simulink model "Controllo_assey_4gdl"  (R2020b)
settings: Solver=VariableStepAuto  StartTime=0.0  StopTime=3  RelTol=1e-3
values from neighbouring files (symbols this model uses):
  my = config_dc(pary)    [mainy.m]
  pary = parametriy ()    [mainy.m]
undefined symbols (not defined in the file or in its folder): accelerazioniy, Evaluate_Trajectory
libraries: cstblocks x4
settings Model: Creator=stefa  LastModifiedBy=user
settings DebuggingCC: SFMachineParentedDataDiag=error

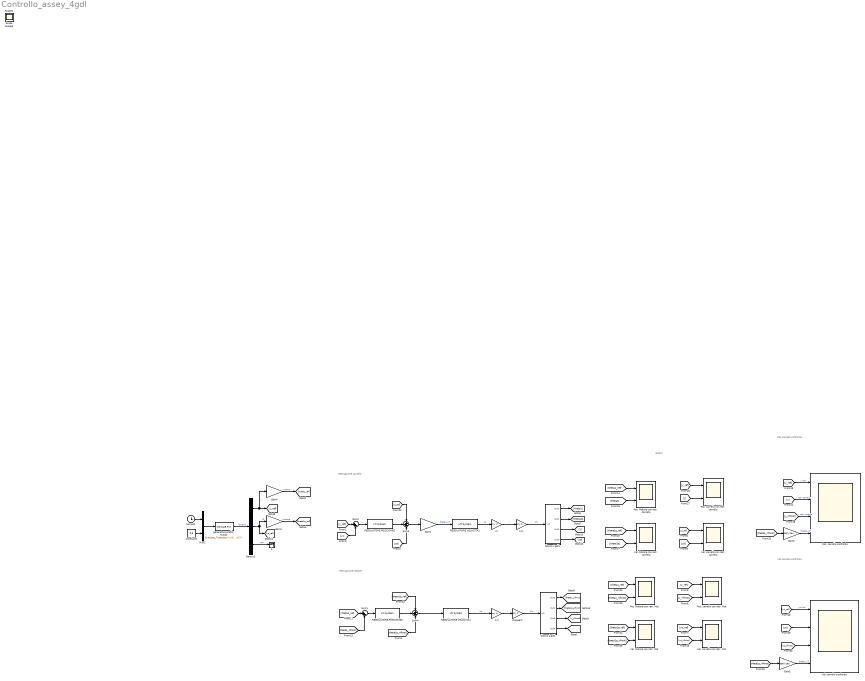
== system Controllo_assey_4gdl ==
  note: Retroazione carrello
  note: Retroazione Motore
  note: Grafici
  note: Pos carrello confronto
  note: Vel carrello confronto
  " 1" : Terminator
  Constant1 : Constant  Value=0.6
  Demux2 : Demux  Outputs=3
  Gain1 : Gain  Gain=1/pary.tau
  Gain2 : Gain  Gain=1/pary.tau
  Gain3 : Gain  Gain=pary.tau
  Gain4 : Gain  Gain=1/pary.tau
  Gain5 : Gain  Gain=pary.tau
  Km : Gain  Gain=my.K
  Kr : Gain  Gain=my.Kr
  Kr1 : Gain  Gain=my.Kr
  Mux1 : Mux  Inputs=2
  Pos. Motore con retr. Mot : Scope  NumInputPorts=2
  Pos. Motore con retr. carrello : Scope  NumInputPorts=2
  Pos. carrello con retr. Mot : Scope  NumInputPorts=2
  Pos. carrello con retr. carrello : Scope  NumInputPorts=2
  Pos. carrello confronto : Scope  NumInputPorts=4
  REGOLATORE POSIZIONE1 : cstblocks/LTI System  sys=ap.H_P  IC=[]
  REGOLATORE POSIZIONE2 : cstblocks/LTI System  sys=ap.H_P  IC=[]
  REGOLATORE VELOCITA1 : cstblocks/LTI System  sys=av.PI_V  IC=[]
  REGOLATORE VELOCITA2 : cstblocks/LTI System  sys=av.PI_V  IC=[]
  Sum1 : Sum  Inputs=|+-
  Sum2 : Sum  Inputs=|+-
  Sum3 : Sum  Inputs=++-
  Sum4 : Sum  Inputs=++-
  Vel. Motore con retr. Mot : Scope  NumInputPorts=2
  Vel. Motore con retr. carrello : Scope  NumInputPorts=2
  Vel. carrello con retr. Mot : Scope  NumInputPorts=2
  Vel. carrello con retr. carrello : Scope  NumInputPorts=2
  Vel. carrello confronto : Scope  NumInputPorts=4
  blocco 4 gdl1 : Subsystem
  blocco 4 gdl2 : Subsystem
  chopper2 : Gain  Gain=my.K
  generatore profilo moto2 : MATLABFcn  MATLABFcn=Evaluate_Trajectory( u(1) , u(2))  OutputDimensions=3
  tempo2 : Clock
  Scope : Scope
  Scope1 : Scope
  Scope3 : Scope
  wires:
  Kr/1 -> Km/1  "I"
  REGOLATORE VELOCITA2/1 -> Kr/1  "Va"
  REGOLATORE POSIZIONE1/1 -> Sum3/2
  Demux2/3 -> " 1"/1  "YPP"
  Mux1/1 -> generatore profilo moto2/1
  generatore profilo moto2/1 -> Demux2/1  "carrello"
  Constant1/1 -> Mux1/2
  [yp_ref] -> Vel. carrello con retr. carrello/1
  [yp] -> Vel. carrello con retr. carrello/2
  [y_ref] -> Pos. carrello con retr. carrello/1
  [y] -> Pos. carrello con retr. carrello/2
  Sum2/1 -> REGOLATORE POSIZIONE1/1
  tempo2/1 -> Mux1/1
  blocco 4 gdl1/3(Out3) -> [y]
  blocco 4 gdl1/4(Out4) -> [yp]
  Km/1 -> blocco 4 gdl1/1(In1)  "Cm"
  Demux2/1 -> [y_ref], Gain4/1  "Y"
  Demux2/2 -> Gain1/1, [yp_ref]  "YP"
  [yp_ref] -> Sum3/1
  Sum3/1 -> Gain2/1
  Gain2/1 -> REGOLATORE VELOCITA2/1  "theta1_rif"
  blocco 4 gdl1/1(Out2) -> [theta1]
  blocco 4 gdl1/2(Out1) -> [theta1p]
  [y_ref] -> Sum2/1
  [y] -> Sum2/2
  [yp] -> Sum3/3
  blocco 4 gdl2/4(Out4) -> [yp_rifmot]
  [y_rifmot] -> Pos. carrello con retr. Mot/2
  chopper2/1 -> blocco 4 gdl2/1(In1)  "Cm"
  blocco 4 gdl2/3(Out3) -> [y_rifmot]
  [theta1_ref] -> Pos. Motore con retr. Mot/1
  Kr1/1 -> chopper2/1  "I"
  Sum1/1 -> REGOLATORE POSIZIONE2/1
  [theta1p_ref] -> Vel. Motore con retr. Mot/1
  REGOLATORE POSIZIONE2/1 -> Sum4/2
  REGOLATORE VELOCITA1/1 -> Kr1/1  "Va"
  blocco 4 gdl2/2(Out1) -> [theta1p_rifmot]
  blocco 4 gdl2/1(Out2) -> [theta1_rifmot]
  [yp_rifmot] -> Vel. carrello con retr. Mot/2
  [yp_ref] -> Vel. carrello con retr. Mot/1
  Sum4/1 -> REGOLATORE VELOCITA1/1
  [y_ref] -> Pos. carrello con retr. Mot/1
  [theta1p_rifmot] -> Vel. Motore con retr. Mot/2
  [theta1_rifmot] -> Pos. Motore con retr. Mot/2
  [theta1p_ref] -> Sum4/1
  Gain4/1 -> [theta1_ref]  "motore"
  [theta1_ref] -> Sum1/1
  Gain1/1 -> [theta1p_ref]  "motore"
  [theta1p_rifmot] -> Sum4/3
  [theta1_rifmot] -> Sum1/2
  [theta1p] -> Vel. Motore con retr. carrello/2
  [theta1] -> Pos. Motore con retr. carrello/2
  [theta1p_ref] -> Vel. Motore con retr. carrello/1
  [theta1_ref] -> Pos. Motore con retr. carrello/1
  [y] -> Pos. carrello confronto/2  "y retr. carrello"
  [y_ref] -> Pos. carrello confronto/1  "y ldm"
  [y_rifmot] -> Pos. carrello confronto/3  "y retr. motore"
  [yp] -> Vel. carrello confronto/2
  [yp_ref] -> Vel. carrello confronto/1  "yp ldm"
  [yp_rifmot] -> Vel. carrello confronto/3
  [theta1_rifmot] -> Gain3/1
  Gain3/1 -> Pos. carrello confronto/4  "theta1_rif"
  [theta1p_rifmot] -> Gain5/1
  Gain5/1 -> Vel. carrello confronto/4  "theta1_rif"

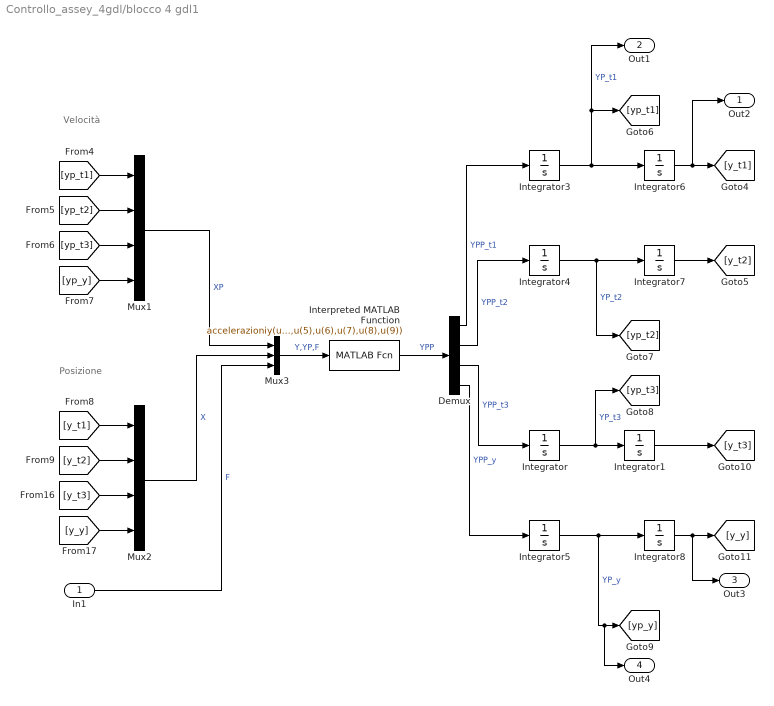
== system Controllo_assey_4gdl/blocco 4 gdl1 ==
  note: Posizione
  note: Velocità
  In1 : Inport
  Demux : Demux
  Integrator{,1,3..7} (7 alike) : Integrator
  Integrator8 : Integrator  InitialCondition=0.0005
  Interpreted MATLAB Function : MATLABFcn  MATLABFcn=accelerazioniy(u(1),u(2),u(3),u(4),u(5),u(6),u(7),u(8),u(9))  OutputDimensions=4
  Mux1 : Mux
  Mux2 : Mux
  Mux3 : Mux  Inputs=3
  Out2 : Outport
  Out1 : Outport  Port=2
  Out3 : Outport  Port=3
  Out4 : Outport  Port=4
  wires:
  Integrator/1 -> Integrator1/1, [yp_t3]  "YP_t3"
  Mux1/1 -> Mux3/1  "XP"
  [y_t3] -> Mux2/3
  Mux3/1 -> Interpreted MATLAB Function/1  "Y,YP,F"
  [y_t2] -> Mux2/2
  Integrator7/1 -> [y_t2]
  Demux/3 -> Integrator/1  "YPP_t3"
  [yp_y] -> Mux1/4
  [y_y] -> Mux2/4
  Demux/1 -> Integrator3/1  "YPP_t1"
  [yp_t2] -> Mux1/2
  Mux2/1 -> Mux3/2  "X"
  Interpreted MATLAB Function/1 -> Demux/1  "YPP"
  Integrator8/1 -> Out3/1, [y_y]
  Integrator4/1 -> [yp_t2], Integrator7/1  "YP_t2"
  Integrator3/1 -> Out1/1, [yp_t1], Integrator6/1  "YP_t1"
  In1/1 -> Mux3/3  "F"
  Demux/2 -> Integrator4/1  "YPP_t2"
  Integrator5/1 -> Out4/1, [yp_y], Integrator8/1  "YP_y"
  Integrator6/1 -> Out2/1, [y_t1]
  [yp_t3] -> Mux1/3
  Demux/4 -> Integrator5/1  "YPP_y"
  Integrator1/1 -> [y_t3]
  [yp_t1] -> Mux1/1
  [y_t1] -> Mux2/1

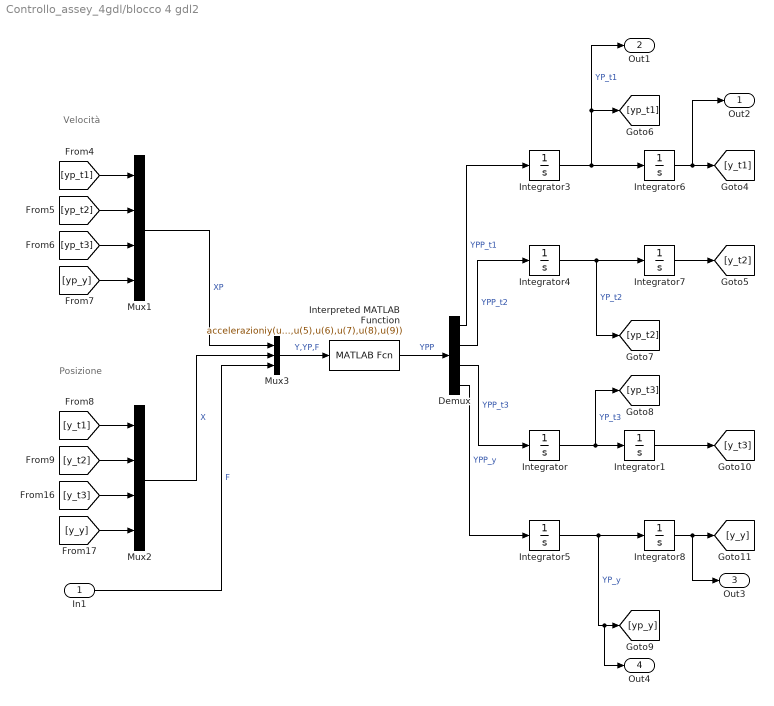
== system Controllo_assey_4gdl/blocco 4 gdl2 ==
  note: Posizione
  note: Velocità
  In1 : Inport
  Demux : Demux
  Integrator{,1,3..7} (7 alike) : Integrator
  Integrator8 : Integrator  InitialCondition=0.0005
  Interpreted MATLAB Function : MATLABFcn  MATLABFcn=accelerazioniy(u(1),u(2),u(3),u(4),u(5),u(6),u(7),u(8),u(9))  OutputDimensions=4
  Mux1 : Mux
  Mux2 : Mux
  Mux3 : Mux  Inputs=3
  Out2 : Outport
  Out1 : Outport  Port=2
  Out3 : Outport  Port=3
  Out4 : Outport  Port=4
  wires:
  Integrator/1 -> Integrator1/1, [yp_t3]  "YP_t3"
  Mux1/1 -> Mux3/1  "XP"
  [y_t3] -> Mux2/3
  Mux3/1 -> Interpreted MATLAB Function/1  "Y,YP,F"
  [y_t2] -> Mux2/2
  Integrator7/1 -> [y_t2]
  Demux/3 -> Integrator/1  "YPP_t3"
  [yp_y] -> Mux1/4
  [y_y] -> Mux2/4
  Demux/1 -> Integrator3/1  "YPP_t1"
  [yp_t2] -> Mux1/2
  Mux2/1 -> Mux3/2  "X"
  Interpreted MATLAB Function/1 -> Demux/1  "YPP"
  Integrator8/1 -> Out3/1, [y_y]
  Integrator4/1 -> [yp_t2], Integrator7/1  "YP_t2"
  Integrator3/1 -> Out1/1, [yp_t1], Integrator6/1  "YP_t1"
  In1/1 -> Mux3/3  "F"
  Demux/2 -> Integrator4/1  "YPP_t2"
  Integrator5/1 -> Out4/1, [yp_y], Integrator8/1  "YP_y"
  Integrator6/1 -> Out2/1, [y_t1]
  [yp_t3] -> Mux1/3
  Demux/4 -> Integrator5/1  "YPP_y"
  Integrator1/1 -> [y_t3]
  [yp_t1] -> Mux1/1
  [y_t1] -> Mux2/1
